simulink model "positiontache"  (R2015b)
settings: Solver=VariableStepAuto  StartTime=0.0  StopTime=10.0  RelTol=1e-3
undefined symbols (not defined in the file or in its folder): G2, Gc, H1
settings Model: Creator=29118  LastModifiedBy=29118

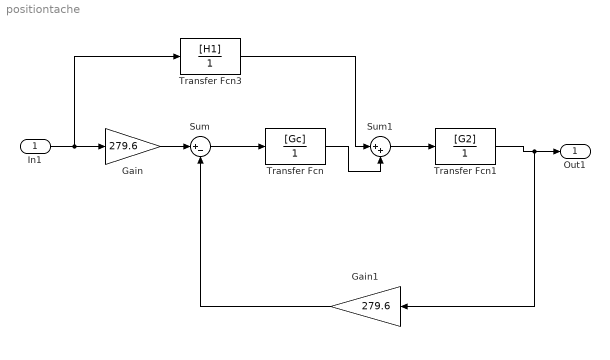
== system positiontache ==
  In1 : Inport
  Gain : Gain  Gain=279.6
  Gain1 : Gain  Gain=279.6
  Sum : Sum  Inputs=|+-
  Sum1 : Sum  Inputs=|++
  Transfer Fcn : TransferFcn  Numerator=[Gc]  Denominator=[ 1]
  Transfer Fcn1 : TransferFcn  Numerator=[G2]  Denominator=[1]
  Transfer Fcn3 : TransferFcn  Numerator=[H1]  Denominator=[1 ]
  Out1 : Outport
  wires:
  Gain/1 -> Sum/1
  Sum/1 -> Transfer Fcn/1
  Sum1/1 -> Transfer Fcn1/1
  Transfer Fcn1/1 -> Gain1/1, Out1/1
  Gain1/1 -> Sum/2
  In1/1 -> Transfer Fcn3/1, Gain/1
  Transfer Fcn/1 -> Sum1/2
  Transfer Fcn3/1 -> Sum1/1
